simulink model "Balashov_LR1"  (R2020b)
settings: Solver=VariableStepAuto  StartTime=0.0  StopTime=0.2  MaxStep=2e-3  RelTol=1e-3
settings Model: Creator=savva  LastModifiedBy=savva

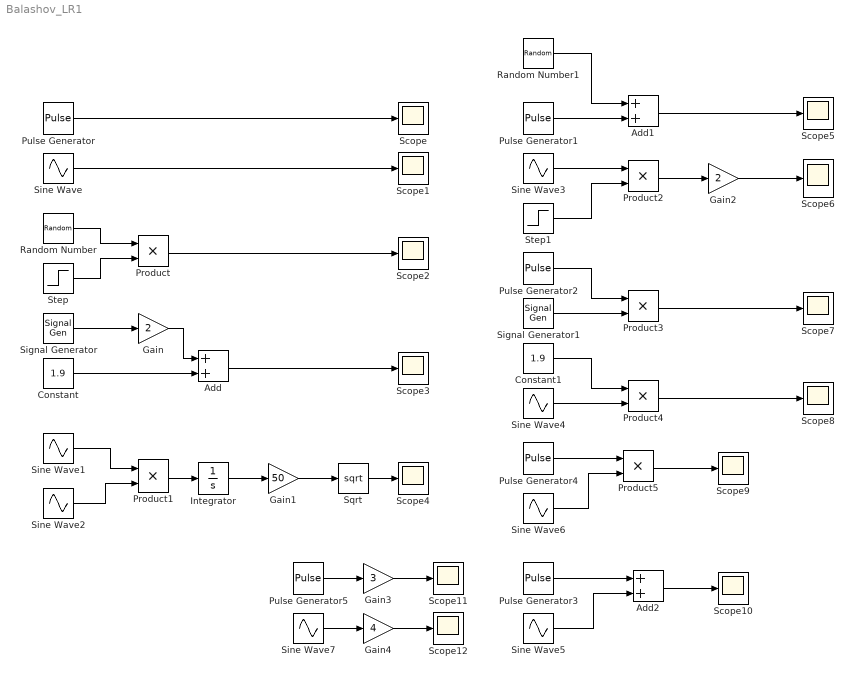
== system Balashov_LR1 ==
  Add : Sum
  Add1 : Sum
  Add2 : Sum
  Constant : Constant  Value=1.9
  Constant1 : Constant  Value=1.9
  Gain : Gain  Gain=2
  Gain1 : Gain  Gain=50
  Gain2 : Gain  Gain=2
  Gain3 : Gain  Gain=3
  Gain4 : Gain  Gain=4
  Integrator : Integrator  UpperSaturationLimit=50  LowerSaturationLimit=0
  Product{,2..5} (5 alike) : Product
  Product1 : Product  CollapseMode=Specified dimension
  Pulse Generator{,1..5} (6 alike) : DiscretePulseGenerator  PulseType=Time based  Amplitude=5  Period=100*10^(-3)  PulseWidth=50
  Random Number : RandomNumber  Mean=2  SampleTime=0.1
  Random Number1 : RandomNumber  Mean=2  SampleTime=0.1
  Scope{,1..12} (13 alike) : Scope
  Signal Generator : SignalGenerator  Amplitude=2  Frequency=100*pi  Units=rad/sec
  Signal Generator1 : SignalGenerator  Amplitude=2  Frequency=100*pi  Units=rad/sec
  Sine Wave{,1..7} (8 alike) : Sin  Amplitude=2  Frequency=100*pi  SampleTime=0
  Sqrt : Sqrt  SaturateOnIntegerOverflow=on
  Step : Step  Time=0.001  SampleTime=0
  Step1 : Step  Time=0.001  SampleTime=0
  wires:
  Pulse Generator/1 -> Scope/1
  Sine Wave/1 -> Scope1/1
  Random Number/1 -> Product/1
  Step/1 -> Product/2
  Product/1 -> Scope2/1
  Signal Generator/1 -> Gain/1
  Gain/1 -> Add/1
  Constant/1 -> Add/2
  Add/1 -> Scope3/1
  Sine Wave1/1 -> Product1/1
  Sine Wave2/1 -> Product1/2
  Product1/1 -> Integrator/1
  Integrator/1 -> Gain1/1
  Gain1/1 -> Sqrt/1
  Sqrt/1 -> Scope4/1
  Random Number1/1 -> Add1/1
  Pulse Generator1/1 -> Add1/2
  Sine Wave3/1 -> Product2/1
  Step1/1 -> Product2/2
  Pulse Generator2/1 -> Product3/1
  Signal Generator1/1 -> Product3/2
  Constant1/1 -> Product4/1
  Sine Wave4/1 -> Product4/2
  Add1/1 -> Scope5/1
  Product3/1 -> Scope7/1
  Product4/1 -> Scope8/1
  Product2/1 -> Gain2/1
  Gain2/1 -> Scope6/1
  Pulse Generator3/1 -> Add2/1
  Sine Wave5/1 -> Add2/2
  Pulse Generator4/1 -> Product5/1
  Sine Wave6/1 -> Product5/2
  Add2/1 -> Scope10/1
  Product5/1 -> Scope9/1
  Pulse Generator5/1 -> Gain3/1
  Sine Wave7/1 -> Gain4/1
  Gain3/1 -> Scope11/1
  Gain4/1 -> Scope12/1
